simulink model "tau_simu_to_xy"  (R2019b)
settings: Solver=VariableStepAuto  StartTime=0.0  StopTime=10.0  FixedStep=0.001  MaxStep=0.2  RelTol=1e-3
settings Model: Creator=kaba  LastModifiedBy=kaba
settings DataIOCC: ExternalInput=[t, u1, u2]  LoadExternalInput=on  SaveFormat=Array  SignalLogging=off  DSMLogging=off

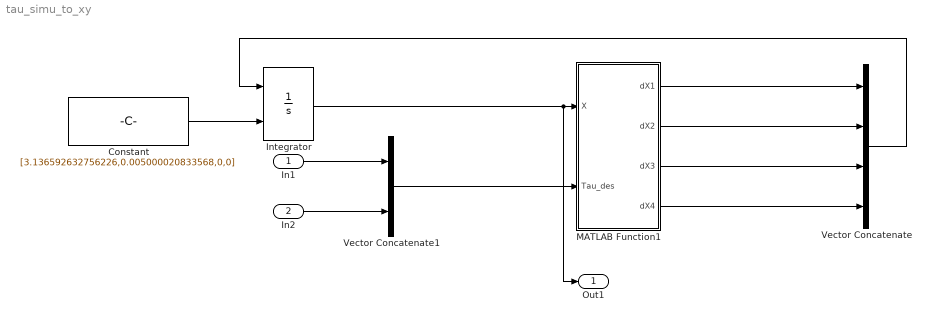
== system tau_simu_to_xy ==
  In1 : Inport
  In2 : Inport  Port=2
  Constant : Constant  Value=[3.136592632756226,0.005000020833568,0,0]
  Integrator : Integrator  InitialConditionSource=external
  MATLAB Function1 : MATLAB Function  TreatAsAtomicUnit=on
  Vector Concatenate : Concatenate  NumInputs=4
  Vector Concatenate1 : Concatenate
  Out1 : Outport
  wires:
  MATLAB Function1/4(dX4) -> Vector Concatenate/4
  MATLAB Function1/1(dX1) -> Vector Concatenate/1
  Vector Concatenate1/1 -> MATLAB Function1/2(Tau_des)
  Constant/1 -> Integrator/2
  Vector Concatenate/1 -> Integrator/1
  MATLAB Function1/3(dX3) -> Vector Concatenate/3
  MATLAB Function1/2(dX2) -> Vector Concatenate/2
  Integrator/1 -> Out1/1, MATLAB Function1/1(X)
  In1/1 -> Vector Concatenate1/1
  In2/1 -> Vector Concatenate1/2

== matlab function tau_simu_to_xy/MATLAB Function1 ==
  data: X input; dX1 output; Tau_des input; dX2 output; dX3 output; dX4 output
function [dX1,dX2,dX3,dX4] = solve_dX(X,Tau_des)

    %% INPUT PARAMETERS
    l1= 1 ;% (m)Length of element 1
    lc1= 0.5 ;%(m) Distance of CM of element 1 from source end
    m1= 6;% (kg) Mass of element 1
    j1= 2;% (kg-m^2) Moment of Inertia of element 1 about its CM

    lc2= 0.5;% (m)Distance of CM of element 2 from source end
    m2= 6;% (kg) Mass of element 2
    j2= 2;% (kg-m^2)Moment of Inertia of element 2 about its CM

    g= 0; % (m/sec^2) Acceleration due to gravity
    
    th1=X(1);
    th2=X(2);
    th1d=X(3);
    th2d=X(4);
    
    %% Simulation Data
    c1=cos(th1);
    c2=cos(th2);
    c21=cos(th2-th1);
    s21=sin(th2-th1);
    
    %%%%%% Dynamic control matrices
    M = [ j1+m2*l1^2, m2*l1*lc2*c21;
          m2*l1*lc2*c21, j2+m2*lc2^2];
    V = [0, -m2*l1*lc2*s21;
        m2*l1*lc2*s21, 0];
    G = [m1*g*lc1*c1+m2*g*l1*c1;
        m2*g*lc2*c2];
    %%%%%%%%%%%%%%%%%%%%%%%%%
    
    %% Generating differential
    [THDD]=M\(Tau_des- V*[th1d^2;th2d^2]-G); %%% Deriving angular acc

    %% Simulation Update
    dX1= th1d;
    dX2= th2d;
    dX3= THDD(1);
    dX4= THDD(2);
